simulink model "untitled1"  (R2023a)
settings: Solver=FixedStepAuto  StartTime=0.0  StopTime=inf  RelTol=1e-3
model workspace (MAT data in the model file):
  SL_ROS_VariableLengthArrays_MaxSizes.CommonInfo.ArrayTruncateAction = 'EmitWarning'
  SL_ROS_VariableLengthArrays_MaxSizes.MsgTypeMap = containers.Map
  SL_ROS_VariableLengthArrays_MaxSizes.MsgTypeMap.serialization.keys = {'diagnostic_msgs/DiagnosticArray', 'diagnostic_msgs/DiagnosticStatus', 'diagnostic_msgs/KeyValue'}
  SL_ROS_VariableLengthArrays_MaxSizes.MsgTypeMap.serialization.values{1}.PropertyName = 'status'
  SL_ROS_VariableLengthArrays_MaxSizes.MsgTypeMap.serialization.values{1}.DataType = 'diagnostic_msgs/DiagnosticStatus'
  SL_ROS_VariableLengthArrays_MaxSizes.MsgTypeMap.serialization.values{1}.MaxLength = 1
  SL_ROS_VariableLengthArrays_MaxSizes.MsgTypeMap.serialization.values{2}(1).PropertyName = 'hardware_id'
  SL_ROS_VariableLengthArrays_MaxSizes.MsgTypeMap.serialization.values{2}(1).DataType = 'uint8'
  SL_ROS_VariableLengthArrays_MaxSizes.MsgTypeMap.serialization.values{2}(1).MaxLength = 128
  SL_ROS_VariableLengthArrays_MaxSizes.MsgTypeMap.serialization.values{2}(2).PropertyName = 'message'
  SL_ROS_VariableLengthArrays_MaxSizes.MsgTypeMap.serialization.values{2}(2).DataType = 'uint8'
  SL_ROS_VariableLengthArrays_MaxSizes.MsgTypeMap.serialization.values{2}(2).MaxLength = 128
  SL_ROS_VariableLengthArrays_MaxSizes.MsgTypeMap.serialization.values{2}(3).PropertyName = 'name'
  SL_ROS_VariableLengthArrays_MaxSizes.MsgTypeMap.serialization.values{2}(3).DataType = 'uint8'
  SL_ROS_VariableLengthArrays_MaxSizes.MsgTypeMap.serialization.values{2}(3).MaxLength = 128
  SL_ROS_VariableLengthArrays_MaxSizes.MsgTypeMap.serialization.values{2}(4).PropertyName = 'values'
  SL_ROS_VariableLengthArrays_MaxSizes.MsgTypeMap.serialization.values{2}(4).DataType = 'diagnostic_msgs/KeyValue'
  SL_ROS_VariableLengthArrays_MaxSizes.MsgTypeMap.serialization.values{2}(4).MaxLength = 3
  SL_ROS_VariableLengthArrays_MaxSizes.MsgTypeMap.serialization.values{3}(1).PropertyName = 'key'
  SL_ROS_VariableLengthArrays_MaxSizes.MsgTypeMap.serialization.values{3}(1).DataType = 'uint8'
  SL_ROS_VariableLengthArrays_MaxSizes.MsgTypeMap.serialization.values{3}(1).MaxLength = 128
  SL_ROS_VariableLengthArrays_MaxSizes.MsgTypeMap.serialization.values{3}(2).PropertyName = 'value'
  SL_ROS_VariableLengthArrays_MaxSizes.MsgTypeMap.serialization.values{3}(2).DataType = 'uint8'
  SL_ROS_VariableLengthArrays_MaxSizes.MsgTypeMap.serialization.values{3}(2).MaxLength = 128
  SL_ROS_VariableLengthArrays_MaxSizes.MsgTypeMap.serialization.uniformity = 0
  SL_ROS_VariableLengthArrays_MaxSizes.MsgTypeMap.serialization.keyType = 'char'
  SL_ROS_VariableLengthArrays_MaxSizes.MsgTypeMap.serialization.valueType = 'any'
undefined symbols (not defined in the file): header, key, key_SL_Info, level, message, message_SL_Info, name, name_SL_Info, status, status_SL_Info, value, value_SL_Info, values, values_SL_Info
libraries: ros2lib x8

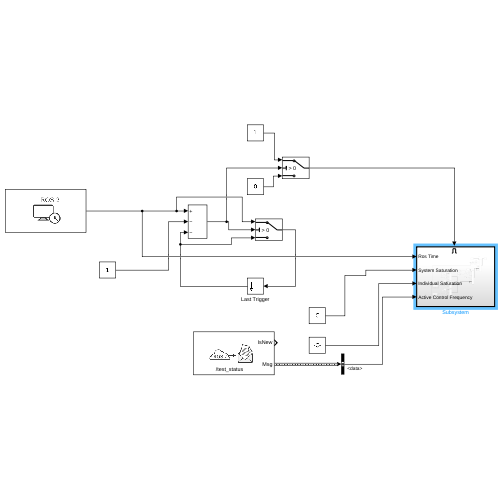
[thumbnail: Simulink's stored preview of the top-level diagram]
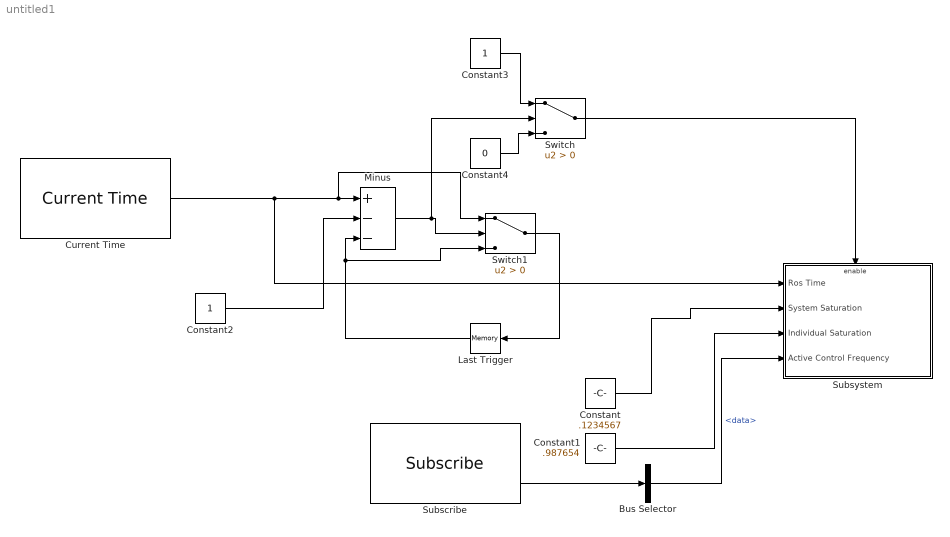
== system untitled1 ==
  Bus Selector : BusSelector  OutputSignals=data
  Constant : Constant  Value=.1234567
  Constant1 : Constant  Value=.987654
  Constant2 : Constant
  Constant3 : Constant
  Constant4 : Constant  Value=0
  Current Time : ros2lib/Current Time  OutputFormat=double  SampleTime=-1  ModelName=untitled1
  Last Trigger : Memory
  Minus : Sum  Inputs=+--
  Subscribe : ros2lib/Subscribe  topicSource=Specify your own  topic=/test_status  messageType=std_msgs/Int8  sampleTime=-1  QOSHistory=Keep last  QOSDepth=1  QOSReliability=Reliable  QOSDurability=Volatile
  Subsystem : Subsystem
  Switch : Switch  Criteria=u2 > Threshold  SaturateOnIntegerOverflow=off  InputSameDT=off
  Switch1 : Switch  Criteria=u2 > Threshold  SaturateOnIntegerOverflow=off  InputSameDT=off
  wires:
  Current Time/1 -> Switch1/1, Minus/1, Subsystem/1(Ros Time)
  Last Trigger/1 -> Switch1/3, Minus/3
  Minus/1 -> Switch/2, Switch1/2
  Switch1/1 -> Last Trigger/1
  Constant2/1 -> Minus/2
  Constant3/1 -> Switch/1
  Constant4/1 -> Switch/3
  Switch/1 -> Subsystem/Enable
  Subscribe/2 -> Bus Selector/1
  Constant/1 -> Subsystem/2(System Saturation)
  Constant1/1 -> Subsystem/3(Individual Saturation)
  Bus Selector/1 -> Subsystem/4(Active Control Frequency)  "<data>"

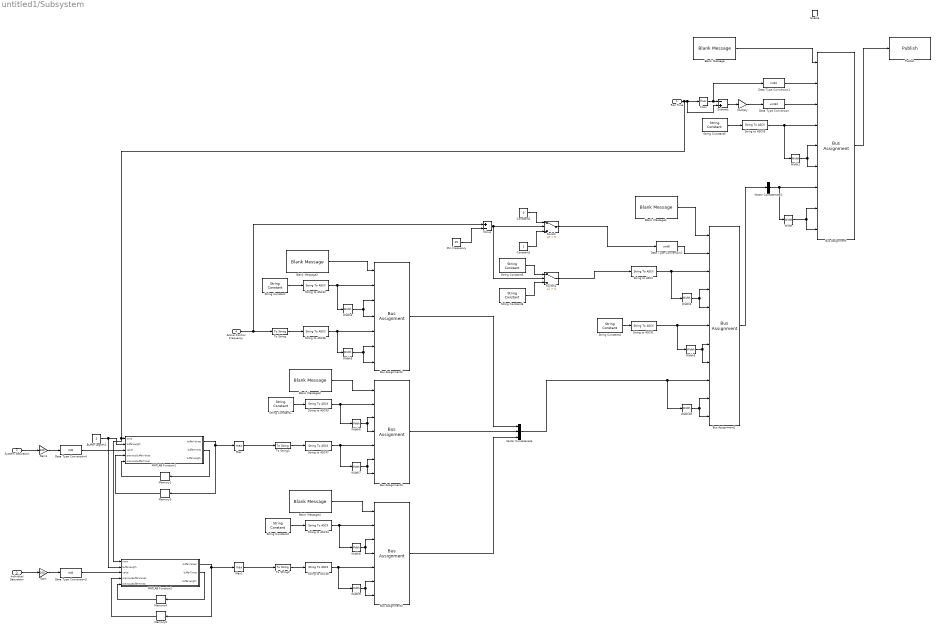
== system untitled1/Subsystem ==
  Ros Time : Inport
  System Saturation : Inport  Port=2
  Individual Saturation : Inport  Port=3
  Active Control Frequency : Inport  Port=4
  Enable : EnablePort
  Blank Message : ros2lib/Blank Message  messageClass=Message  entityType=diagnostic_msgs/DiagnosticArray  messageType=diagnostic_msgs/DiagnosticArray  SampleTime=inf
  Blank Message1 : ros2lib/Blank Message  messageClass=Message  entityType=diagnostic_msgs/DiagnosticStatus  messageType=diagnostic_msgs/DiagnosticStatus  SampleTime=inf
  Blank Message2 : ros2lib/Blank Message  messageClass=Message  entityType=diagnostic_msgs/KeyValue  messageType=diagnostic_msgs/KeyValue  SampleTime=inf
  Blank Message3 : ros2lib/Blank Message  messageClass=Message  entityType=diagnostic_msgs/KeyValue  messageType=diagnostic_msgs/KeyValue  SampleTime=inf
  Blank Message4 : ros2lib/Blank Message  messageClass=Message  entityType=diagnostic_msgs/KeyValue  messageType=diagnostic_msgs/KeyValue  SampleTime=inf
  Buffer Legnth1 : Constant  Value=3
  Bus Assignment : BusAssignment  AssignedSignals=header.stamp.sec,header.stamp.nanosec,header.frame_id,header.frame_id_SL_Info.CurrentLength,header.frame_id_SL_Info.ReceivedLength,status,status_SL_Info.CurrentLength,status_SL_Info.ReceivedLength
  Bus Assignment1 : BusAssignment  AssignedSignals=level,name,name_SL_Info.CurrentLength,name_SL_Info.ReceivedLength,message,message_SL_Info.CurrentLength,message_SL_Info.ReceivedLength,values,values_SL_Info.CurrentLength,values_SL_Info.ReceivedLength
  Bus Assignment2 : BusAssignment  AssignedSignals=key,key_SL_Info.CurrentLength,key_SL_Info.ReceivedLength,value,value_SL_Info.CurrentLength,value_SL_Info.ReceivedLength
  Bus Assignment3 : BusAssignment  AssignedSignals=key,key_SL_Info.CurrentLength,key_SL_Info.ReceivedLength,value,value_SL_Info.CurrentLength,value_SL_Info.ReceivedLength
  Bus Assignment4 : BusAssignment  AssignedSignals=key,key_SL_Info.CurrentLength,key_SL_Info.ReceivedLength,value,value_SL_Info.CurrentLength,value_SL_Info.ReceivedLength
  Constant1 : Constant
  Constant2 : Constant  Value=0
  Data Type Conversion : DataTypeConversion  OutDataTypeStr=uint32  SaturateOnIntegerOverflow=off  RndMeth=Floor
  Data Type Conversion1 : DataTypeConversion  OutDataTypeStr=int32  SaturateOnIntegerOverflow=off  RndMeth=Floor
  Data Type Conversion2 : DataTypeConversion  OutDataTypeStr=uint8  SaturateOnIntegerOverflow=off  RndMeth=Floor
  Data Type Conversion3 : DataTypeConversion  OutDataTypeStr=int8  SaturateOnIntegerOverflow=off  RndMeth=Floor
  Data Type Conversion4 : DataTypeConversion  OutDataTypeStr=int8  SaturateOnIntegerOverflow=off  RndMeth=Floor
  Floor : Rounding
  Gain : Gain  Gain=100
  Gain1 : Gain  Gain=100
  MATLAB Function1 : MATLAB Function  TreatAsAtomicUnit=on
  MATLAB Function2 : MATLAB Function  TreatAsAtomicUnit=on
  Max : MinMax  Function=max
  Max1 : MinMax  Function=max
  Memory{1,3..5} (4 alike) : Memory  InitialCondition=[0,0,0,0,0,0,0,0,0,0,0,0,0,0,0,0,0,0,0,0,0,0,0,0,0,0,0,0,0,0,0,0,0,0,0,0,0,0,0,0,0,0,0,0,0,0,0,0,0,0,0,0,0,0,0,0,0,0,0,0,0,0,0,0,0,0,0,0,0,0,0,0,0,0,0,0,0,0,0,0,0,0,0,0,0,0,0,0,0,0,0,0,0,0,0,0,0,0,0,0,0,0,0,0,0,0,0,0,0,0,0,0,0,0,0,0,0,0,0,0,0,0,0,0,0,0,0,0,0,0,0,0,0,0,0,0,0,0,0,0,0,0,0,0,0,0,0,0,0,0,0,0,0,0,0,0,0,0,0,0,0,0,0,0,0,0,0,0,0,0,0,0,0,0,0,0,0,0,0,0,0,0,0,0,0,0,0,0,0,0,0,0,0,0,0,0,0,0,0,0,0,0,0,0,0,0,0,0,0,0,0,0,0,0,0,0,0,0,0,0,0,0,0,0,0,0,0,0,0,0,0,0,0,0,0,0,0,0,0,0,0,0,0,0,0,0,0,0,0,0,0,0,0,0,0,0]
  Min Frequency : Constant  Value=25
  Minus : Sum  Inputs=+-
  Multiply : Gain  Gain=10^9
  Publish : ros2lib/Publish  topicSource=Specify your own  topic=/diagnostics  messageType=diagnostic_msgs/DiagnosticArray  QOSHistory=Keep last  QOSDepth=1  QOSReliability=Reliable  QOSDurability=Volatile
  String Constant : StringConstant  String="\"Active Control Frequency\""
  String Constant1 : StringConstant  String="\"System Limit Saturation\""
  String Constant2 : StringConstant  String="\"Individual Limit Saturation\""
  String Constant3 : StringConstant  String="\"Complete Controller Operating OK\""
  String Constant4 : StringConstant  String="\"System Status is Represented by Frequency and Saturation Values\""
  String Constant5 : StringConstant  String="\"Complete Controller\""
  String Constant6 : StringConstant  String="\"Complete Controller Operating Slow\""
  String to ASCII{,1..8} (9 alike) : StringToASCII  OutputVectorSize=128
  Subtract : Sum  Inputs=-+
  Switch : Switch  Criteria=u2 > Threshold  SaturateOnIntegerOverflow=off  InputSameDT=off
  Switch1 : Switch  Criteria=u2 > Threshold  SaturateOnIntegerOverflow=off  InputSameDT=off
  To String : ToString
  To String1 : ToString
  To String2 : ToString
  Vector Concatenate : Concatenate  NumInputs=3
  Vector Concatenate1 : Concatenate  NumInputs=1
  Width{,1..10} (11 alike) : Width  DataType=uint32
  wires:
  Blank Message/1 -> Bus Assignment/1
  Bus Assignment/1 -> Publish/1
  Blank Message1/1 -> Bus Assignment1/1
  Bus Assignment1/1 -> Vector Concatenate1/1
  Blank Message2/1 -> Bus Assignment2/1
  String Constant/1 -> String to ASCII2/1
  Active Control Frequency/1 -> Minus/1, To String/1
  String Constant1/1 -> String to ASCII3/1
  Blank Message3/1 -> Bus Assignment3/1
  String Constant2/1 -> String to ASCII4/1
  Blank Message4/1 -> Bus Assignment4/1
  String Constant4/1 -> String to ASCII1/1
  String Constant5/1 -> String to ASCII5/1
  Ros Time/1 -> MATLAB Function2/1(time), MATLAB Function1/1(time), Subtract/2, Floor/1
  Floor/1 -> Data Type Conversion1/1, Subtract/1
  Subtract/1 -> Multiply/1
  Multiply/1 -> Data Type Conversion/1
  String to ASCII/1 -> Width2/1, Bus Assignment1/3
  String to ASCII1/1 -> Width3/1, Bus Assignment1/6
  String to ASCII2/1 -> Width4/1, Bus Assignment2/2
  String to ASCII3/1 -> Width6/1, Bus Assignment3/2
  String to ASCII4/1 -> Width8/1, Bus Assignment4/2
  String to ASCII5/1 -> Width1/1, Bus Assignment/4
  Vector Concatenate/1 -> Width10/1, Bus Assignment1/9
  Bus Assignment3/1 -> Vector Concatenate/2
  Vector Concatenate1/1 -> Width/1, Bus Assignment/7
  To String/1 -> String to ASCII6/1
  String to ASCII6/1 -> Width5/1, Bus Assignment2/5
  To String1/1 -> String to ASCII7/1
  MATLAB Function1/1(bufferValues) -> Max/1, Memory3/1
  String to ASCII7/1 -> Width7/1, Bus Assignment3/5
  To String2/1 -> String to ASCII8/1
  MATLAB Function2/1(bufferValues) -> Max1/1, Memory5/1
  String to ASCII8/1 -> Width9/1, Bus Assignment4/5
  Data Type Conversion/1 -> Bus Assignment/3
  Data Type Conversion1/1 -> Bus Assignment/2
  Width/1 -> Bus Assignment/8, Bus Assignment/9
  Width1/1 -> Bus Assignment/5, Bus Assignment/6
  Width2/1 -> Bus Assignment1/4, Bus Assignment1/5
  Width3/1 -> Bus Assignment1/8, Bus Assignment1/7
  Bus Assignment2/1 -> Vector Concatenate/1
  Bus Assignment4/1 -> Vector Concatenate/3
  Width4/1 -> Bus Assignment2/4, Bus Assignment2/3
  Width5/1 -> Bus Assignment2/7, Bus Assignment2/6
  Width6/1 -> Bus Assignment3/3, Bus Assignment3/4
  Width7/1 -> Bus Assignment3/6, Bus Assignment3/7
  Width8/1 -> Bus Assignment4/4, Bus Assignment4/3
  Width9/1 -> Bus Assignment4/6, Bus Assignment4/7
  Width10/1 -> Bus Assignment1/11, Bus Assignment1/10
  Switch/1 -> Data Type Conversion2/1
  Data Type Conversion2/1 -> Bus Assignment1/2
  Gain1/1 -> Data Type Conversion4/1
  Memory3/1 -> MATLAB Function1/4(previousBufferValues)
  MATLAB Function1/2(bufferTimes) -> Memory1/1
  Memory1/1 -> MATLAB Function1/5(previousBufferTimes)
  Buffer Legnth1/1 -> MATLAB Function2/2("bufferLength "), MATLAB Function1/2("bufferLength ")
  Memory5/1 -> MATLAB Function2/4(previousBufferValues)
  MATLAB Function2/2(bufferTimes) -> Memory4/1
  Memory4/1 -> MATLAB Function2/5(previousBufferTimes)
  Max/1 -> To String1/1
  Max1/1 -> To String2/1
  System Saturation/1 -> Gain1/1
  Individual Saturation/1 -> Gain/1
  Gain/1 -> Data Type Conversion3/1
  Data Type Conversion3/1 -> MATLAB Function2/3(value)
  Data Type Conversion4/1 -> MATLAB Function1/3(value)
  Min Frequency/1 -> Minus/2
  Constant1/1 -> Switch/3
  Constant2/1 -> Switch/1
  Minus/1 -> Switch1/2, Switch/2
  String Constant3/1 -> Switch1/1
  String Constant6/1 -> Switch1/3
  Switch1/1 -> String to ASCII/1

== matlab function untitled1/Subsystem/MATLAB Function1 ==
function [bufferValues, bufferTimes, bufferLength]= bufferValues(time, bufferLength, value, previousBufferValues, previousBufferTimes)

%determine what values to keep in the buffer
%buffer is ordered from newest to oldest
scanning = true;
lastElementToKeep = length(previousBufferTimes) + 1;
lastElementToKeep = min(lastElementToKeep, 256);
while(scanning)
    %increment down
    lastElementToKeep = lastElementToKeep - 1;

    if(lastElementToKeep <= 1 || previousBufferTimes(lastElementToKeep) + bufferLength > time)
        scanning = false;
    end
    
end


bufferValues = zeros(1, 256); 
bufferValues(1) = value;
bufferValues(2:1+lastElementToKeep) = previousBufferValues(1:lastElementToKeep);

bufferTimes = zeros(1, 256);
bufferTimes(1) = time;
bufferTimes(2:1+lastElementToKeep) = previousBufferTimes(1:lastElementToKeep);

bufferLength = (1 + lastElementToKeep);

== matlab function untitled1/Subsystem/MATLAB Function2 ==
function [bufferValues, bufferTimes, bufferLength]= bufferValues(time, bufferLength, value, previousBufferValues, previousBufferTimes)

%determine what values to keep in the buffer
%buffer is ordered from newest to oldest
scanning = true;
lastElementToKeep = length(previousBufferTimes) + 1;
lastElementToKeep = min(lastElementToKeep, 256);
while(scanning)
    %increment down
    lastElementToKeep = lastElementToKeep - 1;

    if(lastElementToKeep <= 1 || previousBufferTimes(lastElementToKeep) + bufferLength > time)
        scanning = false;
    end
    
end


bufferValues = zeros(1, 256); 
bufferValues(1) = value;
bufferValues(2:1+lastElementToKeep) = previousBufferValues(1:lastElementToKeep);

bufferTimes = zeros(1, 256);
bufferTimes(1) = time;
bufferTimes(2:1+lastElementToKeep) = previousBufferTimes(1:lastElementToKeep);

bufferLength = (1 + lastElementToKeep);
